simulink model "SF036A_RtnPahFwl"  (R2013b)
settings: Solver=FixedStepDiscrete  SolverMode=SingleTasking  StartTime=0.0  StopTime=1  FixedStep=0.002  RelTol=1e-3
values from neighbouring files (symbols this model uses):
  ARCHGLBPRM_FLOATZEROTHD_ULS_F32 = DataDict.Constant    [SF036A_RtnPahFwl_DataDict.m]
undefined symbols (not defined in the file or in its folder): MfgEnaSt1, NtcNr1, NtcSts1, sigbuilder_block
libraries: simulink x7, NxtrLim x2, BilnrIntrpnCmnX x2, FixdToFloat x2, FloatToFixdWithRound x1, FloatToFixd x1
Description:
  | This function bounds motor torque commands from SF-02 Active Return, whose primary input is handwheel
  | position.  The incoming motor torque command is saturated to a set of upper and lower boundaries chosen
  | according to handwheel position.
settings Model: CovHTMLOptions=-aTS=1 -bRG=1 -bTC=1 -hTR=0 -nFC=0 -scm=1 -bcm=1 -xEv=0  Creator=lzz0tm  LastModifiedBy=FZG88Y
settings Model: ModifiedHistory=|
  | 001
  | Initial release
  | K. Derry
  | 19-Apr-2012
  | ICR 3358
  | 
  | 002
  | Add logic and display variable to indicate that signal touches boundary.
  | K. Derry
  | 24-Jul-2012
  | ICR-3602
  | 
  | 003
  | Reduce table size and cal only quadrants 1 and 2, calculating 3 and 4.
  | Simplify X-axis boundary to 1-D, no vehicle speed dependency.
  | Add NTC ouput to FDD to match existing code.
  | Eliminate Word doc.
  | K. Derry
  | 23-Jan-2013
  | ICR-3927
  | 
  | 004
  | Add inputs and logic to defeat firewall when SF-02 is defeated.
  | S. Millsap
  | 30-Apr-2013
  | ICR-4102
  | 
  | 005
  | Change Rates and State Execution from Optional to Do Not Execute
  | for Warm Init and from Optional to Execute for Disable
  | S. Millsap
  | 04Dec14
  | ICR-4722
settings SolverCC: AutoInsertRateTranBlk=on  InsertRTBMode=Always
settings DataIOCC: LimitDataPoints=off  SaveFormat=Structure  ReturnWorkspaceOutputs=on
settings OptimizationCC: BlockReduction=off  InlineParams=on  ZeroExternalMemoryAtStartup=off  ZeroInternalMemoryAtStartup=off  OptimizeModelRefInitCode=on  LifeSpan=1
settings DebuggingCC: SignalInfNanChecking=error  SignalRangeChecking=warning  UnderspecifiedInitializationDetection=Simplified  SolverPrmCheckMsg=error  InheritedTsInSrcMsg=error  DiscreteInheritContinuousMsg=error  SingleTaskRateTransMsg=error  TasksWithSamePriorityMsg=error  SigSpecEnsureSampleTimeMsg=error  CheckMatrixSingularityMsg=error  ParameterUnderflowMsg=error  ParameterPrecisionLossMsg=error  ParameterTunabilityLossMsg=error  FixptConstUnderflowMsg=warning  FixptConstOverflowMsg=warning  VectorMatrixConversionMsg=error  SignalLabelMismatchMsg=error  UnconnectedInputMsg=error  UnconnectedOutputMsg=error  UnconnectedLineMsg=error  SFcnCompatibilityMsg=error  UniqueDataStoreMsg=warning  BusObjectLabelMismatch=error  RootOutportRequireBusObject=error  AssertControl=DisableAll  ModelReferenceIOMsg=error  ModelReferenceVersionMismatchMessage=warning  ModelReferenceIOMismatchMessage=error  ModelReferenceCSMismatchMessage=warning  ModelReferenceDataLoggingMessage=error  StateNameClashWarn=warning  StrictBusMsg=ErrorOnBusTreatedAsVector  NonBusSignalsTreatedAsBus=error  SFUnexpectedBacktrackingDiag=error  SFInvalidInputDataAccessInChartInitDiag=error  SFNoUnconditionalDefaultTransitionDiag=error  SFTransitionOutsideNaturalParentDiag=error  SFUnconditionalTransitionShadowingDiag=error  SFUndirectedBroadcastEventsDiag=error
settings ModelReferenceCC: ModelReferenceNumInstancesAllowed=Single
settings RTWCC: SystemTargetFile=autosar.tlc  GenCodeOnly=on  TemplateMakefile=ert_default_tmf  Description=AUTOSAR  GenerateReport=on  ProcessScript=autosar_make_rtw_hook  LaunchReport=on
settings CodeAppCC: GenerateComments=off  IgnoreCustomStorageClasses=off  CustomSymbolStrType=$N$R$M  CustomSymbolStrBlkIO=$N$M  SimulinkBlockComments=off
settings STFCustomTargetCC: ParMdlRefBuildCompliant=on  CompOptLevelCompliant=on  IncludeMdlTerminateFcn=off  CombineOutputUpdateFcns=on  SuppressErrorStatus=on  ERTFirstTimeCompliant=on  ERTCustomFileBanners=on  SupportNonFinite=off  SupportComplex=off  SupportContinuousTime=off  SupportNonInlinedSFcns=off  MATLABClassNameForMDSCustomization=Simulink.SoftwareTarget.ERTCustomization  AutosarCompliant=on  GRTInterface=off  SystemTargetFile=autosar.tlc
settings ERTTargetCC: CodeReplacementLibrary=ANSI_C  ConcurrentExecutionCompliant=off  IncludeMdlTerminateFcn=off  SuppressErrorStatus=on  SupportNonFinite=off  SupportComplex=off  ModelStepFunctionPrototypeControlCompliant=off  CPPClassGenCompliant=off  AutosarCompliant=on  InlinedParameterPlacement=NonHierarchical  ERTCustomFileTemplate=example_file_process.tlc  EnableUserReplacementTypes=on

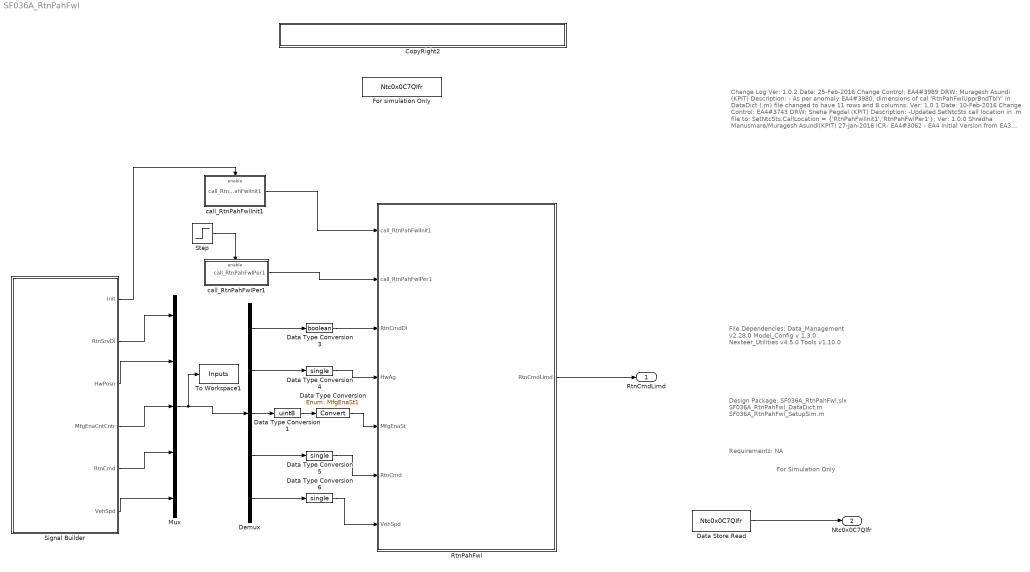
== system SF036A_RtnPahFwl ==
  note: File Dependencies:
      |
      | Data_Management v2.28.0
      | Model_Config v 1.3.0
      | Nexteer_Utilities v4.5.0
      | Tools v1.10.0
  note: Design Package:
      | SF036A_RtnPahFwl.slx
      | SF036A_RtnPahFwl_DataDict.m
      | SF036A_RtnPahFwl_SetupSim.m
  note: Change Log
      |
      | Ver: 1.0.2
      | Date: 25-Feb-2016
      | Change Control: EA4#3989
      | DRW: Muragesh Asundi (KPIT)
      | Description:
      | - As per anomaly EA4#3980, dimensions of cal 'RtnPahFwlUpprBndTblY' in DataDict (.m) file
      | changed to have 11 rows and 8 columns.
      |
      | Ver: 1.0.1
      | Date: 10-Feb-2016
      | Change Control: EA4#3743
      | DRW: Sneha Pegdal (KPIT)
      | Description:
      | -Updated SetNtcSts call location in .m file to:
      |   SetNtcSts.CallLocation = {'RtnPahFwlInit1','RtnPahFwlPer1'};
      |
      | Ver: 1.0.0
      | Shradha Manusmare/Muragesh Asundi(KPIT)
      | 27-Jan-2016
      | ICR- EA4#3062
      | - EA4 Initial Version from EA3 v005
  note: Requirements: NA
  note: For Simulation Only
  CopyRight2 : Subsystem  Description=|  mask(Copyright Information){none=on}
      | Copyright info block.                                               
      |                                                                     
      | Place copyright information at the top of every subsystem in design.
      mask prompts: none "No parameters"
      mask help: Place copyright information at the top of every subsystem in design.
      mask Display:
      | NxtrConf = 'Nexteer Confidential';
      | 
      | sys = bdroot; %handle for the current model ("system")
      | first = get_param(sys,'Created');
      | first = first(end-3:end);  %year is last four digits
      | 
      | last = get_param(sys,'LastModifiedDate');
      | if isempty(last)
      |     last = datestr(now,'yyyy');
      | else
      |     last = last(end-3:end);
      | end
      | 
      | if strcmp(first,last)
      |     fprintf('%s -- Copyright %s Nexteer',NxtrConf,first)
      | else
      |     fprintf('%s -- %s%s- %s Nexteer',NxtrConf,char(169),first,last)
      | end
  Data Store Read : DataStoreRead  DataStoreName=Ntc0x0C7Qlfr  SampleTime=.002
  Data Type Conversion : DataTypeConversion  OutDataTypeStr=Enum: MfgEnaSt1
  Data Type Conversion1 : DataTypeConversion  OutDataTypeStr=uint8
  Data Type Conversion3 : DataTypeConversion  OutDataTypeStr=boolean
  Data Type Conversion4 : DataTypeConversion  OutDataTypeStr=single
  Data Type Conversion5 : DataTypeConversion  OutDataTypeStr=single
  Data Type Conversion6 : DataTypeConversion  OutDataTypeStr=single
  Demux : Demux  Outputs=5
  For simulation Only : DataStoreMemory  DataStoreName=Ntc0x0C7Qlfr  InitialValue=SigQlfr1.SIGQLFR_PASSD  OutDataTypeStr=Enum: SigQlfr1
  Mux : Mux  Inputs=5
  RtnPahFwl : Subsystem
  Signal Builder : Subsystem  Tag=STV Subsys  LoadFcn=sigbuilder_block('load');  StartFcn=sigbuilder_block('start');  StopFcn=sigbuilder_block('stop');  ClipboardFcn=sigbuilder_block('clipboard');  mask(Sigbuilder block){}
      mask help: Simulink:masks:SigbuilderBlock_MD
      mask init:
      | if ~strcmp(get_param(bdroot(gcbh),'SimulationStatus'),'stopped') tuvar = sigbuilder_block('maskInit'); end
      settings: CopyFcn=sigbuilder_block('copy');  DeleteFcn=sigbuilder_block('delete');  ModelCloseFcn=sigbuilder_block('modelClose');  PreSaveFcn=sigbuilder_block('preSave');  PauseFcn=sigbuilder_block('pause');  ContinueFcn=sigbuilder_block('continue');  NameChangeFcn=sigbuilder_block('namechange');  OpenFcn=sigbuilder_block('open',[6 31.5 1012.5 481.5 ]);  CloseFcn=sigbuilder_block('close');
      mask Display: plot(0, 0, 100, 100,[2, 2, 32, 32, 2], [68, 8, 8, 68, 68],[32, 2], [38, 38], [32, 19, 2],[53, 60, 44], [32, 17, 17, 2],[16, 16, 31, 31]);txt = getActiveGroup(gcbh);text(2, 100, txt,'verticalAlignment', 'top');
  Step : Step  SampleTime=0
  To Workspace1 : ToWorkspace  VariableName=Inputs  SampleTime=-1
  call_RtnPahFwlInit1 : Subsystem  TreatAsAtomicUnit=on
  call_RtnPahFwlPer1 : Subsystem
  RtnCmdLimd : Outport
  Ntc0x0C7Qlfr : Outport  Port=2
  wires:
  call_RtnPahFwlInit1/1(call_RtnPahFwlInit1) -> RtnPahFwl/1(call_RtnPahFwlInit1)
  RtnPahFwl/1(RtnCmdLimd) -> RtnCmdLimd/1
  Signal Builder/1(Init) -> call_RtnPahFwlInit1/Enable
  Signal Builder/2(RtnSrvDi) -> Mux/1
  Signal Builder/3(HwPosn) -> Mux/2
  Signal Builder/5(RtnCmd) -> Mux/4
  Signal Builder/6(VehSpd) -> Mux/5
  Demux/1 -> Data Type Conversion3/1
  Demux/2 -> Data Type Conversion4/1
  Demux/4 -> Data Type Conversion5/1
  Data Type Conversion3/1 -> RtnPahFwl/3(RtnCmdDi)
  Data Type Conversion4/1 -> RtnPahFwl/4(HwAg)
  Data Type Conversion5/1 -> RtnPahFwl/6(RtnCmd)
  Data Type Conversion6/1 -> RtnPahFwl/7(VehSpd)
  Demux/5 -> Data Type Conversion6/1
  Mux/1 -> To Workspace1/1, Demux/1
  call_RtnPahFwlPer1/1(call_RtnPahFwlPer1) -> RtnPahFwl/2(call_RtnPahFwlPer1)
  Step/1 -> call_RtnPahFwlPer1/Enable
  Data Store Read/1 -> Ntc0x0C7Qlfr/1
  Demux/3 -> Data Type Conversion1/1
  Data Type Conversion1/1 -> Data Type Conversion/1
  Data Type Conversion/1 -> RtnPahFwl/5(MfgEnaSt)
  Signal Builder/4(MfgEnaCntCntr) -> Mux/3

== system SF036A_RtnPahFwl/CopyRight2 ==

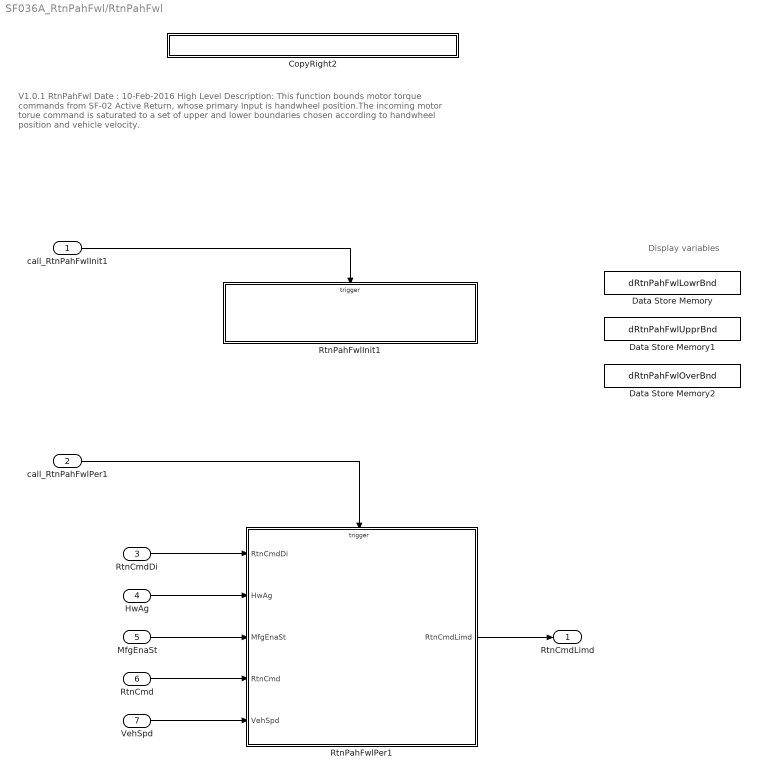
== system SF036A_RtnPahFwl/RtnPahFwl ==
  note: Display variables
  note: V1.0.1    RtnPahFwl                                                                                                          Date : 10-Feb-2016
      |
      | High Level Description:
      |
      | This function bounds motor torque commands from SF-02 Active Return, whose primary Input is handwheel
      | position.The incoming motor torue command is saturated to a set of upper and lower boundaries chosen
      | according to handwheel position and vehicle velocity.
  call_RtnPahFwlInit1 : Inport
  call_RtnPahFwlPer1 : Inport  Port=2
  RtnCmdDi : Inport  Port=3
  HwAg : Inport  Port=4
  MfgEnaSt : Inport  Port=5
  RtnCmd : Inport  Port=6
  VehSpd : Inport  Port=7
  CopyRight2 : Subsystem  Description=|  mask(Copyright Information){none=on}
      | Copyright info block.                                               
      |                                                                     
      | Place copyright information at the top of every subsystem in design.
      mask prompts: none "No parameters"
      mask help: Place copyright information at the top of every subsystem in design.
      mask Display:
      | NxtrConf = 'Nexteer Confidential';
      | 
      | sys = bdroot; %handle for the current model ("system")
      | first = get_param(sys,'Created');
      | first = first(end-3:end);  %year is last four digits
      | 
      | last = get_param(sys,'LastModifiedDate');
      | if isempty(last)
      |     last = datestr(now,'yyyy');
      | else
      |     last = last(end-3:end);
      | end
      | 
      | if strcmp(first,last)
      |     fprintf('%s -- Copyright %s Nexteer',NxtrConf,first)
      | else
      |     fprintf('%s -- %s%s- %s Nexteer',NxtrConf,char(169),first,last)
      | end
  Data Store Memory : DataStoreMemory  DataStoreName=dRtnPahFwlLowrBnd  ReadBeforeWriteMsg=warning  WriteAfterWriteMsg=warning  WriteAfterReadMsg=warning  StateMustResolveToSignalObject=on
  Data Store Memory1 : DataStoreMemory  DataStoreName=dRtnPahFwlUpprBnd  ReadBeforeWriteMsg=warning  WriteAfterWriteMsg=warning  WriteAfterReadMsg=warning  StateMustResolveToSignalObject=on
  Data Store Memory2 : DataStoreMemory  DataStoreName=dRtnPahFwlOverBnd  ReadBeforeWriteMsg=warning  WriteAfterWriteMsg=warning  WriteAfterReadMsg=warning  StateMustResolveToSignalObject=on
  RtnPahFwlInit1 : Subsystem  TreatAsAtomicUnit=on
  RtnPahFwlPer1 : Subsystem
  RtnCmdLimd : Outport
  wires:
  call_RtnPahFwlInit1/1 -> RtnPahFwlInit1/Trigger
  RtnPahFwlPer1/1(RtnCmdLimd) -> RtnCmdLimd/1
  RtnCmdDi/1 -> RtnPahFwlPer1/1(RtnCmdDi)
  HwAg/1 -> RtnPahFwlPer1/2(HwAg)
  MfgEnaSt/1 -> RtnPahFwlPer1/3(MfgEnaSt)
  RtnCmd/1 -> RtnPahFwlPer1/4(RtnCmd)
  VehSpd/1 -> RtnPahFwlPer1/5(VehSpd)
  call_RtnPahFwlPer1/1 -> RtnPahFwlPer1/Trigger

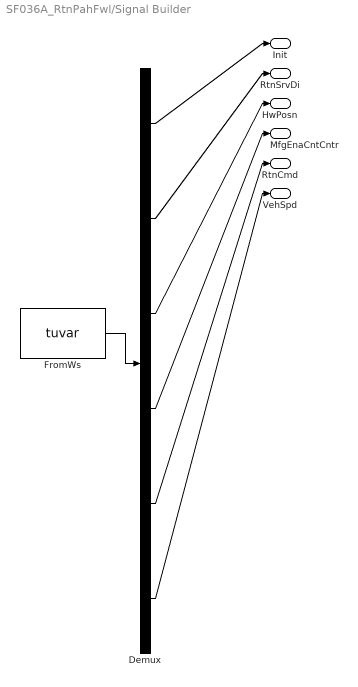
== system SF036A_RtnPahFwl/Signal Builder ==
  Demux : Demux  Tag=STV Demux  Outputs=6
  FromWs : FromWorkspace  Tag=STV FromWs  VariableName=tuvar  SampleTime=0
      SigBuilderData=|
      | common.afterFinalStr = 'Extrapolate'
      | common.sampleTime = 0
      | dataSet.timeRange = [0 0.196]
      | dataSet.name = 'Sheet1'
      | sbobj.Name = 'Signal Builder'
      | sbobj.Groups.Name = 'Sheet1'
      | sbobj.Groups.Signals(1).Name = 'Init'
      | sbobj.Groups.Signals(1).XData = [0 0.002 0.004 0.006 0.008 0.01 0.012 0.014 0.016 0.018 0.02 0.022 0.024 0.026 0.028 0.03 0.032 0.034 0.036 0.038 0.04 0.042 0.044 0.046 0.048 0.05 0.052 0.054 0.056 0.058 0.06 0.062 0.064 0.066 0.068 0.07 0.072 0.074 0.076 0.078 0.08 0.082 0.084 0.086 0.088 0.09 0.092 0.094 0.096 0.098 0.1 0.102 0.104 0.106 0.108 0.11 0.112 0.114 0.116 0.118 0.12 0.122 0.124 0.126 0.128 0.13 0.132 0.134 0.136 0.138 0.14 0.142 0.144 0.146 0.148 0.15 0.152 0.154 0.156 0.158 0.16 0.162 0.164 0.166 0.168 0.17 0.172 0.174 0.176 0.178 0.18 0.182 0.184 0.186 0.188 0.19 0.192 0.194 0.196]
      | sbobj.Groups.Signals(1).YData = [1 0 0 0 0 0 0 0 0 0 0 0 0 0 0 0 0 0 0 0 0 0 0 0 0 0 0 0 0 0 0 0 0 0 0 0 0 0 0 0 0 0 0 0 0 0 0 0 0 0 0 0 0 0 0 0 0 0 0 0 0 0 0 0 0 0 0 0 0 0 0 0 0 0 0 0 0 0 0 0 0 0 0 0 0 0 0 0 0 0 0 0 0 0 0 0 0 0 0]
      | sbobj.Groups.Signals(2).Name = 'RtnSrvDi'
      | sbobj.Groups.Signals(2).XData = [0 0.002 0.004 0.006 0.008 0.01 0.012 0.014 0.016 0.018 0.02 0.022 0.024 0.026 0.028 0.03 0.032 0.034 0.036 0.038 0.04 0.042 0.044 0.046 0.048 0.05 0.052 0.054 0.056 0.058 0.06 0.062 0.064 0.066 0.068 0.07 0.072 0.074 0.076 0.078 0.08 0.082 0.084 0.086 0.088 0.09 0.092 0.094 0.096 0.098 0.1 0.102 0.104 0.106 0.108 0.11 0.112 0.114 0.116 0.118 0.12 0.122 0.124 0.126 0.128 0.13 0.132 0.134 0.136 0.138 0.14 0.142 0.144 0.146 0.148 0.15 0.152 0.154 0.156 0.158 0.16 0.162 0.164 0.166 0.168 0.17 0.172 0.174 0.176 0.178 0.18 0.182 0.184 0.186 0.188 0.19 0.192 0.194 0.196]
      | sbobj.Groups.Signals(2).YData = [0 1 0 1 0 1 0 1 0 1 0 1 0 1 0 1 0 1 0 1 0 1 0 1 0 1 0 1 0 1 0 1 0 1 0 1 0 1 0 1 0 1 0 1 0 1 0 1 0 1 0 1 0 1 0 1 0 1 0 1 0 1 0 1 0 1 0 1 0 1 0 1 0 1 0 1 0 1 0 1 0 1 0 1 0 1 0 1 0 1 0 1 0 1 0 1 0 1 0]
      | sbobj.Groups.Signals(3).Name = 'HwPosn'
      | sbobj.Groups.Signals(3).XData = [0 0.002 0.004 0.006 0.008 0.01 0.012 0.014 0.016 0.018 0.02 0.022 0.024 0.026 0.028 0.03 0.032 0.034 0.036 0.038 0.04 0.042 0.044 0.046 0.048 0.05 0.052 0.054 0.056 0.058 0.06 0.062 0.064 0.066 0.068 0.07 0.072 0.074 0.076 0.078 0.08 0.082 0.084 0.086 0.088 0.09 0.092 0.094 0.096 0.098 0.1 0.102 0.104 0.106 0.108 0.11 0.112 0.114 0.116 0.118 0.12 0.122 0.124 0.126 0.128 0.13 0.132 0.134 0.136 0.138 0.14 0.142 0.144 0.146 0.148 0.15 0.152 0.154 0.156 0.158 0.16 0.162 0.164 0.166 0.168 0.17 0.172 0.174 0.176 0.178 0.18 0.182 0.184 0.186 0.188 0.19 0.192 0.194 0.196]
      | sbobj.Groups.Signals(3).YData = [0.5 72.8518181789 145.020869386 216.824848334 288.082371941 358.613437517 428.239877471 496.785809371 564.078080246 629.946703977 694.225290706 756.751467144 817.367286743 875.91962868 932.26058466 986.247832537 1037.74499584 1086.62198826 1132.75534228 1176.02852103 1216.33221272 1253.56460672 1287.63165078 1318.44728857 1345.93367714 1370.02138347 1390.64955992 1407.76609794 1421.32775966 1431.30028715 1437.65848894 1440.38630365 1439.4768406 1434.93239717 1426.764453 1414.99364105 1399.6496954 1380.77137619 1358.40637169 1332.61117784 1303.45095555 1270.99936607 1235.33838492 1196.55809484 1154.75645821 1110.0390696 1062.518889 1012.31595651 959.557089105 904.375560259 846.910763301 787.307859297 725.717410355 662.294999295 597.20083663 530.599355866 462.658798122 393.550787145 323.449895767 252.533204924 180.979856333 108.97059996 36.6873374384 -35.6873374384 -107.97059996 -179.979856333 -251.533204924 -322.449895767 -392.550787145 -461.658798122 -529.599355866 -596.20083663 -661.294999295 -724.717410355 -786.307859297 -845.910763301 -903.375560259 -958.557089105 -1011.31595651 -1061.518889 -1109.0390696 -1153.75645821 -1195.55809484 -1234.33838492 -1269.99936607 -1302.45095555 -1331.61117784 -1357.40637169 -1379.77137619 -1398.6496954 -1413.99364105 -1425.764453 -1433.93239717 -1438.4768406 -1439.38630365 -1436.65848894 -1430.30028715 -1420.32775966 -1406.76609794]
      | sbobj.Groups.Signals(4).Name = 'MfgEnaCntCntr'
      | sbobj.Groups.Signals(4).XData = [0 0.196]
      | sbobj.Groups.Signals(4).YData = [0 0]
      | sbobj.Groups.Signals(5).Name = 'RtnCmd'
      | sbobj.Groups.Signals(5).XData = [0 0.002 0.004 0.006 0.008 0.01 0.012 0.014 0.016 0.018 0.02 0.022 0.024 0.026 0.028 0.03 0.032 0.034 0.036 0.038 0.04 0.042 0.044 0.046 0.048 0.05 0.052 0.054 0.056 0.058 0.06 0.062 0.064 0.066 0.068 0.07 0.072 0.074 0.076 0.078 0.08 0.082 0.084 0.086 0.088 0.09 0.092 0.094 0.096 0.098 0.1 0.102 0.104 0.106 0.108 0.11 0.112 0.114 0.116 0.118 0.12 0.122 0.124 0.126 0.128 0.13 0.132 0.134 0.136 0.138 0.14 0.142 0.144 0.146 0.148 0.15 0.152 0.154 0.156 0.158 0.16 0.162 0.164 0.166 0.168 0.17 0.172 0.174 0.176 0.178 0.18 0.182 0.184 0.186 0.188 0.19 0.192 0.194 0.196]
      | sbobj.Groups.Signals(5).YData = [0.5 0.942149999982 1.38318309069 1.82198518426 2.25744782853 2.68847100705 3.11396591788 3.53285772394 3.94408826817 4.34661874653 4.7394323321 5.12153674366 5.49196675232 5.84978661971 6.19409246181 6.52401453217 6.83871941901 7.13741215048 7.4193382028 7.68378540631 7.93008574442 8.15761704109 8.36580453253 8.55412231906 8.72209469362 8.8692973434 8.99535842173 9.0999594874 9.18283630903 9.24377953258 9.28263521017 9.29930518899 9.29374735924 9.26597576046 9.21606054613 9.14412780641 9.05035924965 8.93499174335 8.79831671586 8.64067942014 8.4624780617 8.26416279263 8.0462345745 7.80924391292 7.55378946686 7.28051653643 6.99011543275 6.68331973423 6.36090443342 6.02368397936 5.67251022017 5.30827025126 4.93188417439 4.54430277347 4.14650511274 3.73949606363 3.3243037663 2.90197703255 2.47358269635 2.04020291898 1.60293245537 1.16287588865 0.721144839901 0.278855160099 -0.162875888646 -0.602932455366 -1.04020291898 -1.47358269635 -1.90197703255 -2.3243037663 -2.73949606363 -3.14650511274 -3.54430277347 -3.93188417439 -4.30827025126 -4.67251022017 -5.02368397936 -5.36090443342 -5.68331973423 -5.99011543275 -6.28051653643 -6.55378946686 -6.80924391292 -7.0462345745 -7.26416279263 -7.4624780617 -7.64067942014 -7.79831671586 -7.93499174335 -8.05035924965 -8.14412780641 -8.21606054613 -8.26597576046 -8.29374735924 -8.29930518899 -8.28263521017 -8.24377953258 -8.18283630903 -8.0999594874]
      | sbobj.Groups.Signals(6).Name = 'VehSpd'
      | sbobj.Groups.Signals(6).XData = [0 0.002 0.004 0.006 0.008 0.01 0.012 0.014 0.016 0.018 0.02 0.022 0.024 0.026 0.028 0.03 0.032 0.034 0.036 0.038 0.04 0.042 0.044 0.046 0.048 0.05 0.052 0.054 0.056 0.058 0.06 0.062 0.064 0.066 0.068 0.07 0.072 0.074 0.076 0.078 0.08 0.082 0.084 0.086 0.088 0.09 0.092 0.094 0.096 0.098 0.1 0.102 0.104 0.106 0.108 0.11 0.112 0.114 0.116 0.118 0.12 0.122 0.124 0.126 0.128 0.13 0.132 0.134 0.136 0.138 0.14 0.142 0.144 0.146 0.148 0.15 0.152 0.154 0.156 0.158 0.16 0.162 0.164 0.166 0.168 0.17 0.172 0.174 0.176 0.178 0.18 0.182 0.184 0.186 0.188 0.19 0.192 0.194 0.196]
      | sbobj.Groups.Signals(6).YData = [0.5 26.1748465899 51.784836289 77.2652760407 102.551800043 127.580532341 152.288248186 176.612533742 200.491943754 223.866156759 246.676127466 268.86423591 290.374433004 311.152382122 331.145596362 350.30357113 368.577911718 385.922455556 402.293388822 417.649357116 431.951569932 445.163898636 457.252967741 468.188239209 477.942089595 486.489879827 493.810017444 499.884011143 504.69651749 508.235379676 510.491658227 511.459653588 511.136920519 509.524274272 506.625788531 502.448785122 497.003815519 490.304634188 482.368163841 473.214452692 462.86662381 451.350816708 438.696121315 424.934504489 410.100729269 394.232267058 377.36920297 359.554134567 340.832064259 321.25028562 300.858263921 279.707511181 257.851456036 235.345308778 212.245921888 188.611646422 164.502184611 139.978439049 115.102358845 89.9367831364 64.5452823514 38.9919976248 13.3414787715 0.5 26.1748465899 51.784836289 77.2652760407 102.551800043 127.580532341 152.288248186 176.612533742 200.491943754 223.866156759 246.676127466 268.86423591 290.374433004 311.152382122 331.145596362 350.30357113 368.577911718 385.922455556 402.293388822 417.649357116 431.951569932 445.163898636 457.252967741 468.188239209 477.942089595 486.489879827 493.810017444 499.884011143 504.69651749 508.235379676 510.491658227 511.459653588 511.136920519 509.524274272 506.625788531 502.448785122]
      | sbobj.Groups.TimeRange = [0 0.196]
  Init : Outport
  RtnSrvDi : Outport  Tag=STV Outport  Port=2
  HwPosn : Outport  Tag=STV Outport  Port=3
  MfgEnaCntCntr : Outport  Tag=STV Outport  Port=4
  RtnCmd : Outport  Tag=STV Outport  Port=5
  VehSpd : Outport  Tag=STV Outport  Port=6
  wires:
  FromWs/1 -> Demux/1
  Demux/1 -> Init/1
  Demux/2 -> RtnSrvDi/1
  Demux/3 -> HwPosn/1
  Demux/4 -> MfgEnaCntCntr/1
  Demux/5 -> RtnCmd/1
  Demux/6 -> VehSpd/1

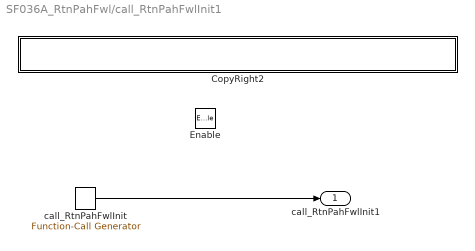
== system SF036A_RtnPahFwl/call_RtnPahFwlInit1 ==
  Enable : EnablePort
  CopyRight2 : Subsystem  Description=|  mask(Copyright Information){none=on}
      | Copyright info block.                                               
      |                                                                     
      | Place copyright information at the top of every subsystem in design.
      mask prompts: none "No parameters"
      mask help: Place copyright information at the top of every subsystem in design.
      mask Display:
      | NxtrConf = 'Nexteer Confidential';
      | 
      | sys = bdroot; %handle for the current model ("system")
      | first = get_param(sys,'Created');
      | first = first(end-3:end);  %year is last four digits
      | 
      | last = get_param(sys,'LastModifiedDate');
      | if isempty(last)
      |     last = datestr(now,'yyyy');
      | else
      |     last = last(end-3:end);
      | end
      | 
      | if strcmp(first,last)
      |     fprintf('%s -- Copyright %s Nexteer',NxtrConf,first)
      | else
      |     fprintf('%s -- %s%s- %s Nexteer',NxtrConf,char(169),first,last)
      | end
  "call_RtnPahFwlInit " : simulink/Ports & Subsystems/Function-Call Generator  sample_time=0  numberOfIterations=1
  call_RtnPahFwlInit1 : Outport
  wires:
  "call_RtnPahFwlInit "/1 -> call_RtnPahFwlInit1/1

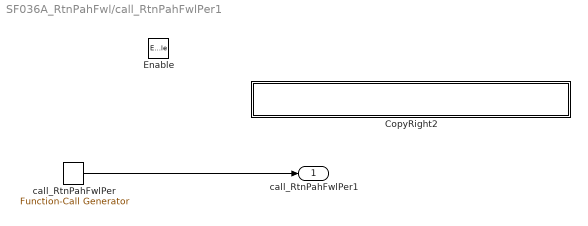
== system SF036A_RtnPahFwl/call_RtnPahFwlPer1 ==
  Enable : EnablePort
  CopyRight2 : Subsystem  Description=|  mask(Copyright Information){none=on}
      | Copyright info block.                                               
      |                                                                     
      | Place copyright information at the top of every subsystem in design.
      mask prompts: none "No parameters"
      mask help: Place copyright information at the top of every subsystem in design.
      mask Display:
      | NxtrConf = 'Nexteer Confidential';
      | 
      | sys = bdroot; %handle for the current model ("system")
      | first = get_param(sys,'Created');
      | first = first(end-3:end);  %year is last four digits
      | 
      | last = get_param(sys,'LastModifiedDate');
      | if isempty(last)
      |     last = datestr(now,'yyyy');
      | else
      |     last = last(end-3:end);
      | end
      | 
      | if strcmp(first,last)
      |     fprintf('%s -- Copyright %s Nexteer',NxtrConf,first)
      | else
      |     fprintf('%s -- %s%s- %s Nexteer',NxtrConf,char(169),first,last)
      | end
  call_RtnPahFwlPer : simulink/Ports & Subsystems/Function-Call Generator  sample_time=0.002  numberOfIterations=1
  call_RtnPahFwlPer1 : Outport
  wires:
  call_RtnPahFwlPer/1 -> call_RtnPahFwlPer1/1

== system SF036A_RtnPahFwl/RtnPahFwl/CopyRight2 ==

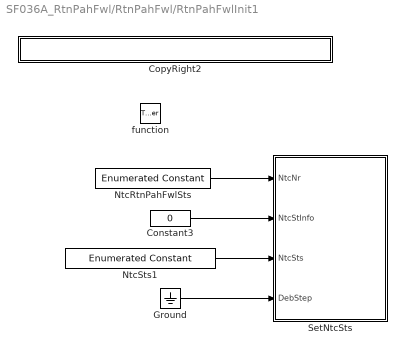
== system SF036A_RtnPahFwl/RtnPahFwl/RtnPahFwlInit1 ==
  function : TriggerPort  TriggerType=function-call
  Constant3 : Constant  Value=0  OutDataTypeStr=uint8
      settings: AttributesFormatString=%<OutDataTypeStr>
  CopyRight2 : Subsystem  Description=|  mask(Copyright Information){none=on}
      | Copyright info block.                                               
      |                                                                     
      | Place copyright information at the top of every subsystem in design.
      mask prompts: none "No parameters"
      mask help: Place copyright information at the top of every subsystem in design.
      mask Display:
      | NxtrConf = 'Nexteer Confidential';
      | 
      | sys = bdroot; %handle for the current model ("system")
      | first = get_param(sys,'Created');
      | first = first(end-3:end);  %year is last four digits
      | 
      | last = get_param(sys,'LastModifiedDate');
      | if isempty(last)
      |     last = datestr(now,'yyyy');
      | else
      |     last = last(end-3:end);
      | end
      | 
      | if strcmp(first,last)
      |     fprintf('%s -- Copyright %s Nexteer',NxtrConf,first)
      | else
      |     fprintf('%s -- %s%s- %s Nexteer',NxtrConf,char(169),first,last)
      | end
  Ground : Ground
  NtcRtnPahFwlSts : simulink/Sources/Enumerated Constant  OutDataTypeStr=Enum: NtcNr1  Value=NtcNr1.NTCNR_0X0C7  SampleTime=inf
  NtcSts1 : simulink/Sources/Enumerated Constant  OutDataTypeStr=Enum: NtcSts1  Value=NtcSts1.NTCSTS_PASSD  SampleTime=inf
  SetNtcSts : Subsystem  mask(SetNTC){}
      mask help: SetNTC library block
  wires:
  NtcRtnPahFwlSts/1 -> SetNtcSts/1(NtcNr)
  Constant3/1 -> SetNtcSts/2(NtcStInfo)
  NtcSts1/1 -> SetNtcSts/3(NtcSts)
  Ground/1 -> SetNtcSts/4(DebStep)

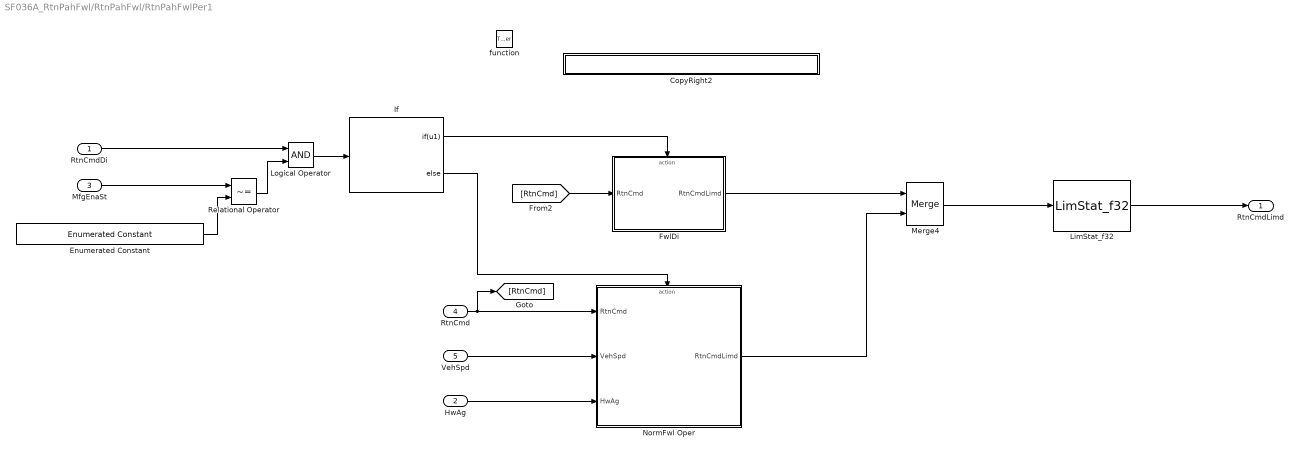
== system SF036A_RtnPahFwl/RtnPahFwl/RtnPahFwlPer1 ==
  RtnCmdDi : Inport
  HwAg : Inport  Port=2
  MfgEnaSt : Inport  Port=3
  RtnCmd : Inport  Port=4
  VehSpd : Inport  Port=5
  function : TriggerPort  TriggerType=function-call
  CopyRight2 : Subsystem  Description=|  mask(Copyright Information){none=on}
      | Copyright info block.                                               
      |                                                                     
      | Place copyright information at the top of every subsystem in design.
      mask prompts: none "No parameters"
      mask help: Place copyright information at the top of every subsystem in design.
      mask Display:
      | NxtrConf = 'Nexteer Confidential';
      | 
      | sys = bdroot; %handle for the current model ("system")
      | first = get_param(sys,'Created');
      | first = first(end-3:end);  %year is last four digits
      | 
      | last = get_param(sys,'LastModifiedDate');
      | if isempty(last)
      |     last = datestr(now,'yyyy');
      | else
      |     last = last(end-3:end);
      | end
      | 
      | if strcmp(first,last)
      |     fprintf('%s -- Copyright %s Nexteer',NxtrConf,first)
      | else
      |     fprintf('%s -- %s%s- %s Nexteer',NxtrConf,char(169),first,last)
      | end
  Enumerated Constant : simulink/Sources/Enumerated Constant  OutDataTypeStr=Enum: MfgEnaSt1  Value=MfgEnaSt1.MFGENAST_PRDNMOD  SampleTime=-1
  FwlDi : Subsystem  TreatAsAtomicUnit=on
  If : If  IfExpression=u1
  LimStat_f32 : NxtrLim/LimStat_f32  LoLim=SYSGLBPRM_MOTTQCMDLOLIM_MOTNWTMTR_F32  HiLim=SYSGLBPRM_MOTTQCMDHILIM_MOTNWTMTR_F32
      settings: AttributesFormatString=|
      | Low Limit: %<LoLim>
      | High Limit:%<HiLim>
  Logical Operator : Logic  AllPortsSameDT=off  OutDataTypeStr=boolean
  Merge4 : Merge
  NormFwl Oper : Subsystem  TreatAsAtomicUnit=on
  Relational Operator : RelationalOperator  Operator=~=  OutDataTypeStr=boolean
  RtnCmdLimd : Outport
  wires:
  VehSpd/1 -> NormFwl Oper/2(VehSpd)
  HwAg/1 -> NormFwl Oper/3(HwAg)
  RtnCmd/1 -> [RtnCmd], NormFwl Oper/1(RtnCmd)
  If/1 -> FwlDi/Action
  [RtnCmd] -> FwlDi/1(RtnCmd)
  NormFwl Oper/1(RtnCmdLimd) -> Merge4/2
  If/2 -> NormFwl Oper/Action
  FwlDi/1(RtnCmdLimd) -> Merge4/1
  RtnCmdDi/1 -> Logical Operator/1
  Relational Operator/1 -> Logical Operator/2
  Logical Operator/1 -> If/1
  Merge4/1 -> LimStat_f32/1
  LimStat_f32/1 -> RtnCmdLimd/1
  Enumerated Constant/1 -> Relational Operator/2
  MfgEnaSt/1 -> Relational Operator/1

== system SF036A_RtnPahFwl/call_RtnPahFwlInit1/CopyRight2 ==

== system SF036A_RtnPahFwl/call_RtnPahFwlPer1/CopyRight2 ==

== system SF036A_RtnPahFwl/RtnPahFwl/RtnPahFwlInit1/CopyRight2 ==

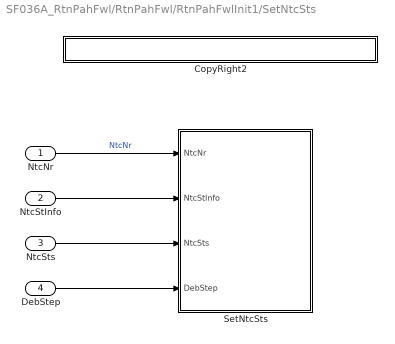
== system SF036A_RtnPahFwl/RtnPahFwl/RtnPahFwlInit1/SetNtcSts ==
  NtcNr : Inport
  NtcStInfo : Inport  Port=2
  NtcSts : Inport  Port=3
  DebStep : Inport  Port=4
  CopyRight2 : Subsystem  Description=|  mask(Copyright Information){none=on}
      | Copyright info block.                                               
      |                                                                     
      | Place copyright information at the top of every subsystem in design.
      mask prompts: none "No parameters"
      mask help: Place copyright information at the top of every subsystem in design.
      mask Display:
      | NxtrConf = 'Nexteer Confidential';
      | 
      | sys = bdroot; %handle for the current model ("system")
      | first = get_param(sys,'Created');
      | first = first(end-3:end);  %year is last four digits
      | 
      | last = get_param(sys,'LastModifiedDate');
      | if isempty(last)
      |     last = datestr(now,'yyyy');
      | else
      |     last = last(end-3:end);
      | end
      | 
      | if strcmp(first,last)
      |     fprintf('%s -- Copyright %s Nexteer',NxtrConf,first)
      | else
      |     fprintf('%s -- %s%s- %s Nexteer',NxtrConf,char(169),first,last)
      | end
  SetNtcSts : Subsystem  RequirementInfo={} %GIDa_f357c891_c5a6_41fb_bb31_ba5af47c5b52  TreatAsAtomicUnit=on
      settings: RTWSystemCode=Inline
  wires:
  NtcNr/1 -> SetNtcSts/1(NtcNr)  "NtcNr"
  NtcSts/1 -> SetNtcSts/3(NtcSts)
  DebStep/1 -> SetNtcSts/4(DebStep)
  NtcStInfo/1 -> SetNtcSts/2(NtcStInfo)

== system SF036A_RtnPahFwl/RtnPahFwl/RtnPahFwlPer1/CopyRight2 ==

== system SF036A_RtnPahFwl/RtnPahFwl/RtnPahFwlPer1/FwlDi ==
  RtnCmd : Inport
  Action Port : ActionPort  ActionType=then
  CopyRight2 : Subsystem  Description=|  mask(Copyright Information){none=on}
      | Copyright info block.                                               
      |                                                                     
      | Place copyright information at the top of every subsystem in design.
      mask prompts: none "No parameters"
      mask help: Place copyright information at the top of every subsystem in design.
      mask Display:
      | NxtrConf = 'Nexteer Confidential';
      | 
      | sys = bdroot; %handle for the current model ("system")
      | first = get_param(sys,'Created');
      | first = first(end-3:end);  %year is last four digits
      | 
      | last = get_param(sys,'LastModifiedDate');
      | if isempty(last)
      |     last = datestr(now,'yyyy');
      | else
      |     last = last(end-3:end);
      | end
      | 
      | if strcmp(first,last)
      |     fprintf('%s -- Copyright %s Nexteer',NxtrConf,first)
      | else
      |     fprintf('%s -- %s%s- %s Nexteer',NxtrConf,char(169),first,last)
      | end
  RtnCmdLimd : Outport
  wires:
  RtnCmd/1 -> RtnCmdLimd/1

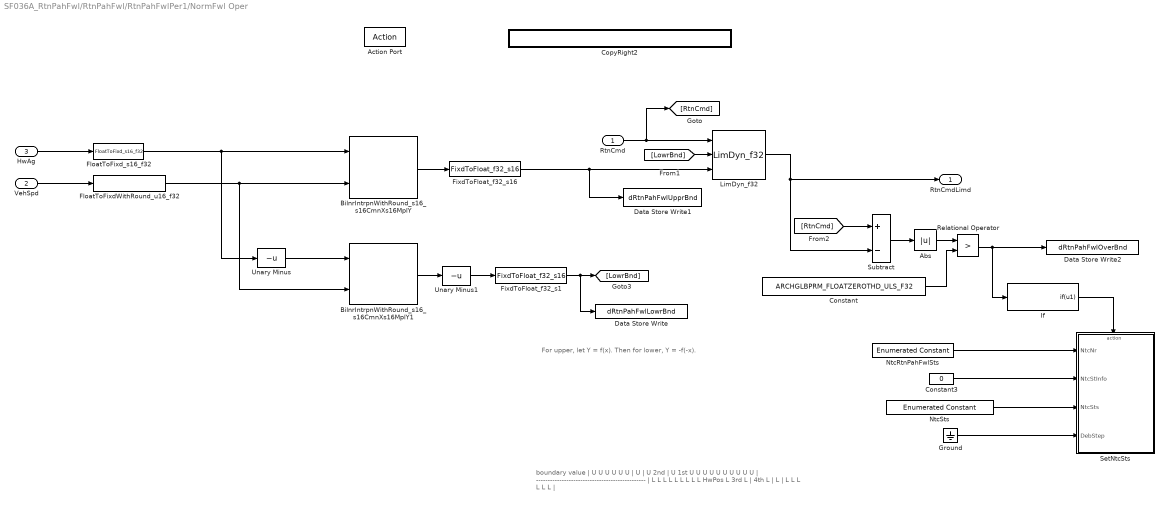
== system SF036A_RtnPahFwl/RtnPahFwl/RtnPahFwlPer1/NormFwl Oper ==
  note: boundary value
      |                    |       U U U U U U
      |                    |     U
      |                    |   U
      |       2nd          | U       1st
      |                    U
      |  U U U U U U U U U |
      | -----------------------------------------------
      |                    | L L L L L L L L L    HwPos
      |                    L
      |       3rd        L |         4th
      |                L   |
      |              L     |
      |  L L L L L L       |
  note: For upper, let Y = f(x). Then for lower, Y = -f(-x).
  RtnCmd : Inport
  VehSpd : Inport  Port=2
  HwAg : Inport  Port=3
  Action Port : ActionPort  ActionType=else
  Abs : Abs
  BilnrIntrpnWithRound_s16_s16CmnXs16MplY : BilnrIntrpnCmnX/BilnrIntrpnWithRound_s16_s16CmnXs16MplY  XTbl=RtnPahFwlUpprBndTblX  MplYTbl=RtnPahFwlUpprBndTblY  BilnrSelnTbl=RtnPahFwlVehSpd
      settings: AttributesFormatString=Bilnr ( s16CmnX , s16MplY )
  BilnrIntrpnWithRound_s16_s16CmnXs16MplY1 : BilnrIntrpnCmnX/BilnrIntrpnWithRound_s16_s16CmnXs16MplY  XTbl=RtnPahFwlUpprBndTblX  MplYTbl=RtnPahFwlUpprBndTblY  BilnrSelnTbl=RtnPahFwlVehSpd
      settings: AttributesFormatString=Bilnr ( s16CmnX , s16MplY )
  Constant : Constant  Value=ARCHGLBPRM_FLOATZEROTHD_ULS_F32
  Constant3 : Constant  Value=0  OutDataTypeStr=uint8
      settings: AttributesFormatString=%<OutDataTypeStr>
  CopyRight2 : Subsystem  Description=|  mask(Copyright Information){none=on}
      | Copyright info block.                                               
      |                                                                     
      | Place copyright information at the top of every subsystem in design.
      mask prompts: none "No parameters"
      mask help: Place copyright information at the top of every subsystem in design.
      mask Display:
      | NxtrConf = 'Nexteer Confidential';
      | 
      | sys = bdroot; %handle for the current model ("system")
      | first = get_param(sys,'Created');
      | first = first(end-3:end);  %year is last four digits
      | 
      | last = get_param(sys,'LastModifiedDate');
      | if isempty(last)
      |     last = datestr(now,'yyyy');
      | else
      |     last = last(end-3:end);
      | end
      | 
      | if strcmp(first,last)
      |     fprintf('%s -- Copyright %s Nexteer',NxtrConf,first)
      | else
      |     fprintf('%s -- %s%s- %s Nexteer',NxtrConf,char(169),first,last)
      | end
  Data Store Write : DataStoreWrite  DataStoreName=dRtnPahFwlLowrBnd
  Data Store Write1 : DataStoreWrite  DataStoreName=dRtnPahFwlUpprBnd
  Data Store Write2 : DataStoreWrite  DataStoreName=dRtnPahFwlOverBnd
  FixdToFloat_f32_s1 : FixdToFloat/FixdToFloat_f32_s16  Param1=11
  FixdToFloat_f32_s16 : FixdToFloat/FixdToFloat_f32_s16  Param1=11
  FloatToFixdWithRound_u16_f32 : FloatToFixdWithRound/FloatToFixdWithRound_u16_f32  Param1=7
  FloatToFixd_s16_f32 : FloatToFixd/FloatToFixd_s16_f32  Param1=4
  Ground : Ground
  If : If  IfExpression=u1  ShowElse=off
  LimDyn_f32 : NxtrLim/LimDyn_f32
  NtcRtnPahFwlSts : simulink/Sources/Enumerated Constant  OutDataTypeStr=Enum: NtcNr1  Value=NtcNr1.NTCNR_0X0C7  SampleTime=inf
  NtcSts : simulink/Sources/Enumerated Constant  OutDataTypeStr=Enum: NtcSts1  Value=NtcSts1.NTCSTS_FAILD  SampleTime=inf
  Relational Operator : RelationalOperator  Operator=>  OutDataTypeStr=boolean
  SetNtcSts : Subsystem  mask(SetNTC){}
      mask help: SetNTC library block
  Subtract : Sum  Inputs=+-
  Unary Minus : UnaryMinus
  Unary Minus1 : UnaryMinus
  RtnCmdLimd : Outport
  wires:
  [LowrBnd] -> LimDyn_f32/2
  HwAg/1 -> FloatToFixd_s16_f32/1
  Unary Minus1/1 -> FixdToFloat_f32_s1/1
  FixdToFloat_f32_s1/1 -> Data Store Write/1, [LowrBnd]
  FloatToFixd_s16_f32/1 -> Unary Minus/1, BilnrIntrpnWithRound_s16_s16CmnXs16MplY/1
  VehSpd/1 -> FloatToFixdWithRound_u16_f32/1
  BilnrIntrpnWithRound_s16_s16CmnXs16MplY/1 -> FixdToFloat_f32_s16/1
  FixdToFloat_f32_s16/1 -> Data Store Write1/1, LimDyn_f32/3
  RtnCmd/1 -> [RtnCmd], LimDyn_f32/1
  LimDyn_f32/1 -> Subtract/2, RtnCmdLimd/1
  [RtnCmd] -> Subtract/1
  Unary Minus/1 -> BilnrIntrpnWithRound_s16_s16CmnXs16MplY1/1
  FloatToFixdWithRound_u16_f32/1 -> BilnrIntrpnWithRound_s16_s16CmnXs16MplY1/2, BilnrIntrpnWithRound_s16_s16CmnXs16MplY/2
  BilnrIntrpnWithRound_s16_s16CmnXs16MplY1/1 -> Unary Minus1/1
  Subtract/1 -> Abs/1
  Abs/1 -> Relational Operator/1
  Relational Operator/1 -> If/1, Data Store Write2/1
  Constant/1 -> Relational Operator/2
  NtcRtnPahFwlSts/1 -> SetNtcSts/1(NtcNr)
  Ground/1 -> SetNtcSts/4(DebStep)
  Constant3/1 -> SetNtcSts/2(NtcStInfo)
  NtcSts/1 -> SetNtcSts/3(NtcSts)
  If/1 -> SetNtcSts/Action

== system SF036A_RtnPahFwl/RtnPahFwl/RtnPahFwlInit1/SetNtcSts/CopyRight2 ==

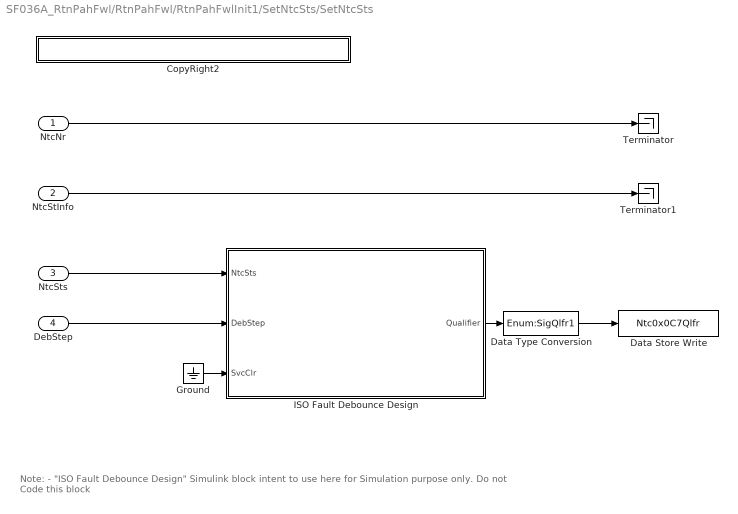
== system SF036A_RtnPahFwl/RtnPahFwl/RtnPahFwlInit1/SetNtcSts/SetNtcSts ==
  note: Note:
      |
      | - "ISO Fault Debounce Design" Simulink block intent to use here for Simulation purpose only. Do not Code this block
  NtcNr : Inport
  NtcStInfo : Inport  Port=2
  NtcSts : Inport  Port=3
  DebStep : Inport  Port=4
  CopyRight2 : Subsystem  Description=|  mask(Copyright Information){none=on}
      | Copyright info block.                                               
      |                                                                     
      | Place copyright information at the top of every subsystem in design.
      mask prompts: none "No parameters"
      mask help: Place copyright information at the top of every subsystem in design.
      mask Display:
      | NxtrConf = 'Nexteer Confidential';
      | 
      | sys = bdroot; %handle for the current model ("system")
      | first = get_param(sys,'Created');
      | first = first(end-3:end);  %year is last four digits
      | 
      | last = get_param(sys,'LastModifiedDate');
      | if isempty(last)
      |     last = datestr(now,'yyyy');
      | else
      |     last = last(end-3:end);
      | end
      | 
      | if strcmp(first,last)
      |     fprintf('%s -- Copyright %s Nexteer',NxtrConf,first)
      | else
      |     fprintf('%s -- %s%s- %s Nexteer',NxtrConf,char(169),first,last)
      | end
  Data Store Write : DataStoreWrite  DataStoreName=Ntc0x0C7Qlfr
  Data Type Conversion : DataTypeConversion  OutDataTypeStr=Enum:SigQlfr1
  Ground : Ground
  ISO Fault Debounce Design : Stateflow chart  TreatAsAtomicUnit=on
      settings: AttributesFormatString=|
      | Simulation Purpose Only.
      | Do Not Code this block
      | Diagnostic Manager Owns this requirement
  Terminator : Terminator
  Terminator1 : Terminator
  wires:
  NtcStInfo/1 -> Terminator1/1
  NtcNr/1 -> Terminator/1
  NtcSts/1 -> ISO Fault Debounce Design/1(NtcSts)
  DebStep/1 -> ISO Fault Debounce Design/2(DebStep)
  ISO Fault Debounce Design/1(Qualifier) -> Data Type Conversion/1
  Ground/1 -> ISO Fault Debounce Design/3(SvcClr)
  Data Type Conversion/1 -> Data Store Write/1

== system SF036A_RtnPahFwl/RtnPahFwl/RtnPahFwlPer1/FwlDi/CopyRight2 ==

== system SF036A_RtnPahFwl/RtnPahFwl/RtnPahFwlPer1/NormFwl Oper/CopyRight2 ==

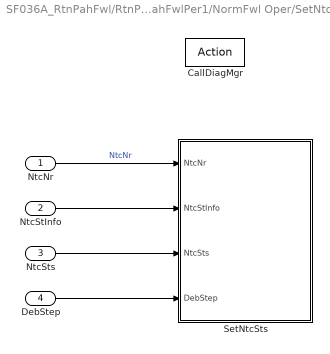
== system SF036A_RtnPahFwl/RtnPahFwl/RtnPahFwlPer1/NormFwl Oper/SetNtcSts ==
  NtcNr : Inport
  NtcStInfo : Inport  Port=2
  NtcSts : Inport  Port=3
  DebStep : Inport  Port=4
  CallDiagMgr : ActionPort  ActionType=then
  SetNtcSts : Subsystem  RequirementInfo={} %GIDa_4c387ebe_8ad4_4b50_b2e0_2b1bca063896  TreatAsAtomicUnit=on
      settings: RTWSystemCode=Inline
  wires:
  NtcStInfo/1 -> SetNtcSts/2(NtcStInfo)
  DebStep/1 -> SetNtcSts/4(DebStep)
  NtcSts/1 -> SetNtcSts/3(NtcSts)
  NtcNr/1 -> SetNtcSts/1(NtcNr)  "NtcNr"

== system SF036A_RtnPahFwl/RtnPahFwl/RtnPahFwlInit1/SetNtcSts/SetNtcSts/CopyRight2 ==

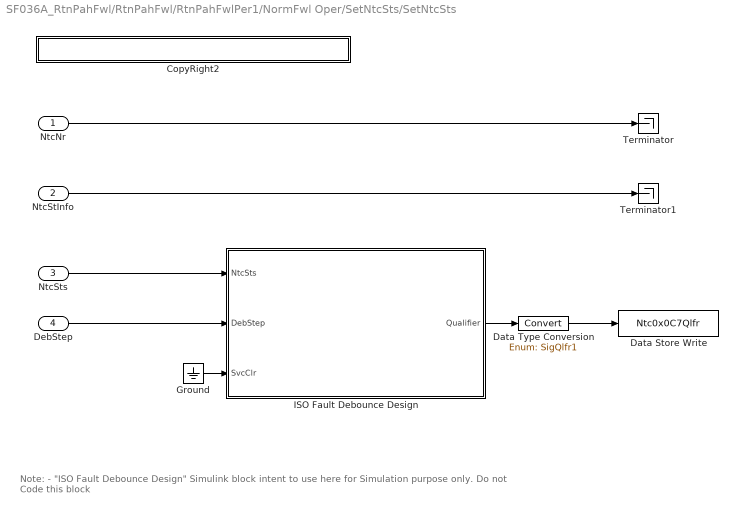
== system SF036A_RtnPahFwl/RtnPahFwl/RtnPahFwlPer1/NormFwl Oper/SetNtcSts/SetNtcSts ==
  note: Note:
      |
      | - "ISO Fault Debounce Design" Simulink block intent to use here for Simulation purpose only. Do not Code this block
  NtcNr : Inport
  NtcStInfo : Inport  Port=2
  NtcSts : Inport  Port=3
  DebStep : Inport  Port=4
  CopyRight2 : Subsystem  Description=|  mask(Copyright Information){none=on}
      | Copyright info block.                                               
      |                                                                     
      | Place copyright information at the top of every subsystem in design.
      mask prompts: none "No parameters"
      mask help: Place copyright information at the top of every subsystem in design.
      mask Display:
      | NxtrConf = 'Nexteer Confidential';
      | 
      | sys = bdroot; %handle for the current model ("system")
      | first = get_param(sys,'Created');
      | first = first(end-3:end);  %year is last four digits
      | 
      | last = get_param(sys,'LastModifiedDate');
      | if isempty(last)
      |     last = datestr(now,'yyyy');
      | else
      |     last = last(end-3:end);
      | end
      | 
      | if strcmp(first,last)
      |     fprintf('%s -- Copyright %s Nexteer',NxtrConf,first)
      | else
      |     fprintf('%s -- %s%s- %s Nexteer',NxtrConf,char(169),first,last)
      | end
  Data Store Write : DataStoreWrite  DataStoreName=Ntc0x0C7Qlfr
  Data Type Conversion : DataTypeConversion  OutDataTypeStr=Enum: SigQlfr1
  Ground : Ground
  ISO Fault Debounce Design : Stateflow chart  TreatAsAtomicUnit=on
      settings: AttributesFormatString=|
      | Simulation Purpose Only.
      | Do Not Code this block
      | Diagnostic Manager Owns this requirement
  Terminator : Terminator
  Terminator1 : Terminator
  wires:
  Ground/1 -> ISO Fault Debounce Design/3(SvcClr)
  ISO Fault Debounce Design/1(Qualifier) -> Data Type Conversion/1
  DebStep/1 -> ISO Fault Debounce Design/2(DebStep)
  NtcSts/1 -> ISO Fault Debounce Design/1(NtcSts)
  NtcNr/1 -> Terminator/1
  NtcStInfo/1 -> Terminator1/1
  Data Type Conversion/1 -> Data Store Write/1

== system SF036A_RtnPahFwl/RtnPahFwl/RtnPahFwlPer1/NormFwl Oper/SetNtcSts/SetNtcSts/CopyRight2 ==

== stateflow chart SF036A_RtnPahFwl/RtnPahFwl/RtnPahFwlPer1/NormFwl Oper/SetNtcSts/SetNtcSts/ISO Fault Debounce Design ==
  note: NTCSTS_PASSD           (0)
      | NTCSTS_FAILD             (1)
      | NTCSTS_PREPASSD   (2)
      | NTCSTS_PREFAILD     (3)
      |
      | SIGQLFR_NORES        (0)
      | SIGQLFR_PASSD         (1)
      | SIGQLFR_FAILD           (2)
  note: Pass Loop
  note: Fail Loop
  note: 
  (default) -> (junction 89)
  (junction 89) -> (junction 95) [order 1] : [NtcSts ==3]
  (junction 89) -> (junction 93) [order 2] : [NtcSts ==2]
  (junction 89) -> (junction 141) [order 3] : [NtcSts ==1]
      | { ErrAcc = 32767;
      | Qualifier =2;
      |  }
  (junction 89) -> (junction 141) [order 4] : [NtcSts ==0]
      | { ErrAcc = -32768;
      | Qualifier=1;
      | }
  (junction 95) -> (junction 103) [order 2]
  (junction 95) -> (junction 111) [order 1] : [ErrAcc <=0]
      | {ErrAcc = DebStep;}
  (junction 93) -> (junction 123) [order 2] : {
      | ErrAcc = ErrAcc - DebStep;
      | }
  (junction 93) -> (junction 123) [order 1] : [(ErrAcc - DebStep) <= -32768]
      | { ErrAcc = -32768;
      | Qualifier=1;
      | }
  (junction 103) -> (junction 111) [order 1] : [(ErrAcc + DebStep) <32767]
      | {ErrAcc = ErrAcc + DebStep;}
  (junction 103) -> (junction 111) [order 2] : {ErrAcc = 32767;
      | Qualifier =2;}
  (junction 123) -> (junction 141)
  (junction 111) -> (junction 141)
  (junction 141) -> (junction 159) [order 2] : {ErrAcc = 0;
      | Qualifier =0;
      | }
  (junction 141) -> (junction 159) [order 1] : [SvcClr ==0]
  data: NtcSts input Enum: NtcSts1; Qualifier output uint8; DebStep input uint16; ErrAcc local single; SvcClr input

== stateflow chart SF036A_RtnPahFwl/RtnPahFwl/RtnPahFwlInit1/SetNtcSts/SetNtcSts/ISO Fault Debounce Design ==
  note: NTCSTS_PASSD           (0)
      | NTCSTS_FAILD             (1)
      | NTCSTS_PREPASSD   (2)
      | NTCSTS_PREFAILD     (3)
      |
      | SIGQLFR_NORES        (0)
      | SIGQLFR_PASSD         (1)
      | SIGQLFR_FAILD           (2)
  note: Pass Loop
  note: Fail Loop
  note: 
  (default) -> (junction 89)
  (junction 89) -> (junction 95) [order 1] : [NtcSts ==3]
  (junction 89) -> (junction 93) [order 2] : [NtcSts ==2]
  (junction 89) -> (junction 141) [order 3] : [NtcSts ==1]
      | { ErrAcc = 32767;
      | Qualifier =2;
      |  }
  (junction 89) -> (junction 141) [order 4] : [NtcSts ==0]
      | { ErrAcc = -32768;
      | Qualifier=1;
      | }
  (junction 95) -> (junction 103) [order 2]
  (junction 95) -> (junction 111) [order 1] : [ErrAcc <=0]
      | {ErrAcc = DebStep;}
  (junction 93) -> (junction 123) [order 2] : {
      | ErrAcc = ErrAcc - DebStep;
      | }
  (junction 93) -> (junction 123) [order 1] : [(ErrAcc - DebStep) <= -32768]
      | { ErrAcc = -32768;
      | Qualifier=1;
      | }
  (junction 103) -> (junction 111) [order 1] : [(ErrAcc + DebStep) <32767]
      | {ErrAcc = ErrAcc + DebStep;}
  (junction 103) -> (junction 111) [order 2] : {ErrAcc = 32767;
      | Qualifier =2;}
  (junction 123) -> (junction 141)
  (junction 111) -> (junction 141)
  (junction 141) -> (junction 159) [order 2] : {ErrAcc = 0;
      | Qualifier =0;
      | }
  (junction 141) -> (junction 159) [order 1] : [SvcClr ==0]
  data: NtcSts input Enum: NtcSts1; Qualifier output uint8; DebStep input uint16; ErrAcc local single; SvcClr input
